simulink model "tp2p2demo"  (R2015a)
settings: Solver=ode45  StartTime=0.0  StopTime=10.0  RelTol=1e-3
values from neighbouring files (symbols this model uses):
  a = 1    [Untitled.m]
  am = 2    [Untitled.m]
  b = .5    (= 0.5)    [Untitled.m]
  bm = 2    [Untitled.m]
  t1 = bm / b    (= 4)    [Untitled.m]
  t2 = (am - a) / b    (= 2)    [Untitled.m]
settings Model: Creator=Dano  LastModifiedBy=Dano

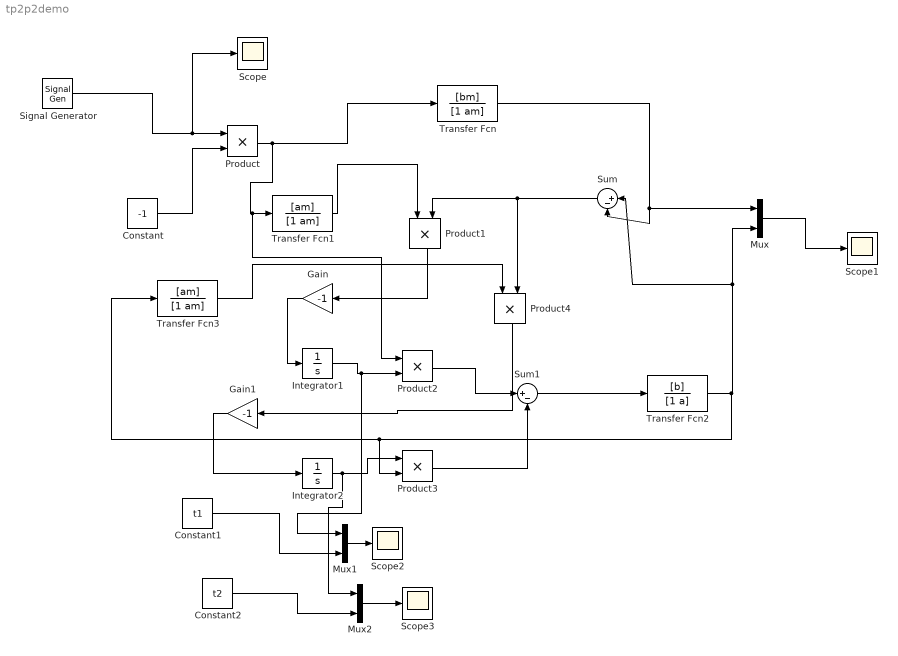
== system tp2p2demo ==
  Constant : Constant  Value=-1
  Constant1 : Constant  Value=t1
  Constant2 : Constant  Value=t2
  Gain : Gain  Gain=-1
  Gain1 : Gain  Gain=-1
  Integrator1 : Integrator
  Integrator2 : Integrator
  Mux : Mux  Inputs=2
  Mux1 : Mux  Inputs=2
  Mux2 : Mux  Inputs=2
  Product{,1..4} (5 alike) : Product
  Scope{,1..3} (4 alike) : Scope
      Scope2 settings: SaveName=ScopeData2
      Scope3 settings: SaveName=ScopeData3
  Signal Generator : SignalGenerator  WaveForm=square  Frequency=1/20  Units=rad/sec
  Sum : Sum  Inputs=|+-
  Sum1 : Sum  Inputs=|+-
  Transfer Fcn : TransferFcn  Numerator=[bm]  Denominator=[1 am]
  Transfer Fcn1 : TransferFcn  Numerator=[am]  Denominator=[1 am]
  Transfer Fcn2 : TransferFcn  Numerator=[b]  Denominator=[1 a]
  Transfer Fcn3 : TransferFcn  Numerator=[am]  Denominator=[1 am]
  wires:
  Constant/1 -> Product/2
  Signal Generator/1 -> Scope/1, Product/1
  Product/1 -> Product2/1, Transfer Fcn1/1, Transfer Fcn/1
  Transfer Fcn1/1 -> Product1/1
  Product1/1 -> Gain/1
  Gain/1 -> Integrator1/1
  Integrator1/1 -> Mux1/1, Product2/2
  Product2/1 -> Sum1/1
  Product3/1 -> Sum1/2
  Sum1/1 -> Transfer Fcn2/1
  Transfer Fcn3/1 -> Product4/1
  Transfer Fcn/1 -> Mux/1, Sum/2
  Sum/1 -> Product4/2, Product1/2
  Product4/1 -> Gain1/1
  Gain1/1 -> Integrator2/1
  Integrator2/1 -> Mux2/1, Product3/1
  Transfer Fcn2/1 -> Transfer Fcn3/1, Product3/2, Mux/2, Sum/1
  Mux/1 -> Scope1/1
  Mux2/1 -> Scope3/1
  Mux1/1 -> Scope2/1
  Constant1/1 -> Mux1/2
  Constant2/1 -> Mux2/2
